simulink model "Appl_DrMotorAdjust_CtrlModel"  (R2018b)
settings: configuration reference "CodeConfig_10_ms" (kept outside this file)
undefined symbols (not defined in the file): CAL_HightMotorRunInterval_100ms, CAL_MotorDiffToStart_100ms, CAL_MotorStopTime_50ms, D_Relay_DownBackFault, D_Relay_UpFrontFault, D_ToleranceDistance, enSeatMoveCmd, FALSE, TRUE
libraries: DareLib x88, simulink x2
(part 1 of 3)
settings Model: Creator=Administrator  LastModifiedBy=Administrator
settings ConfigSetRef: SourceLocation=Base Workspace

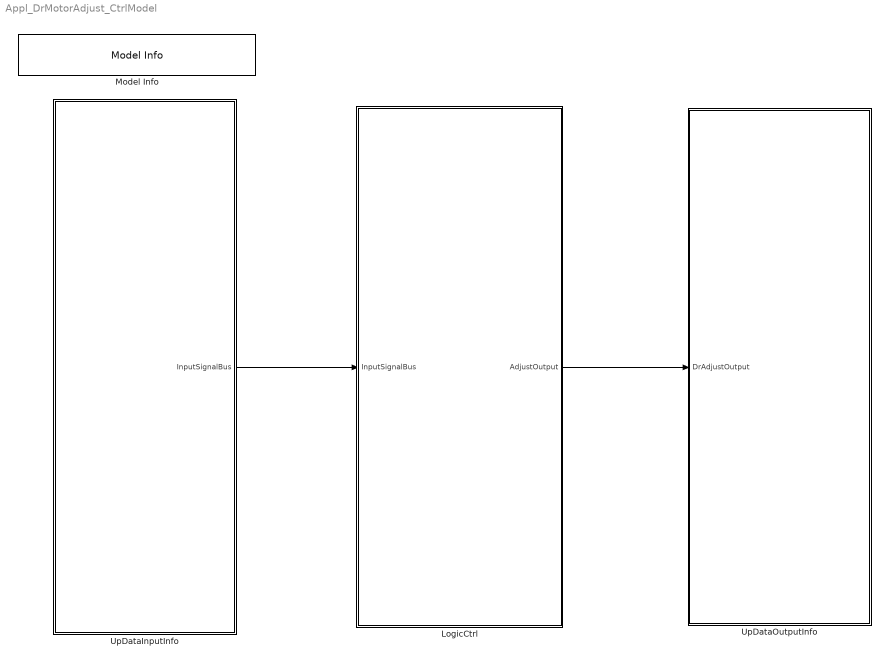
== system Appl_DrMotorAdjust_CtrlModel ==
  LogicCtrl : Subsystem  Priority=2  TreatAsAtomicUnit=on
      settings: RTWSystemCode=Nonreusable function  RTWFcnNameOpts=Use subsystem name
  Model Info : simulink/Model-Wide Utilities/Model Info  Frame=on  DisplayStringWithTags=Version：%<ModelVersion>  HorizontalTextAlignment=Center  LeftAlignmentValue=0.5
  UpDataInputInfo : Subsystem  Priority=1  TreatAsAtomicUnit=on
      settings: RTWSystemCode=Nonreusable function  RTWFcnNameOpts=Use subsystem name
  UpDataOutputInfo : Subsystem  Priority=3  TreatAsAtomicUnit=on
      settings: RTWSystemCode=Nonreusable function  RTWFcnNameOpts=Use subsystem name
  wires:
  UpDataInputInfo/1(InputSignalBus) -> LogicCtrl/1(InputSignalBus)
  LogicCtrl/1(AdjustOutput) -> UpDataOutputInfo/1(DrAdjustOutput)

== system Appl_DrMotorAdjust_CtrlModel/LogicCtrl ==
  InputSignalBus : Inport
  LocalAdjustCtrl : Subsystem  Description=调节逻辑处理
      settings: AttributesFormatString=%<Description>
  AdjustOutput : Outport
  wires:
  InputSignalBus/1 -> LocalAdjustCtrl/1(RteInputBus)  "RteInputBus"
  LocalAdjustCtrl/1(LocalAdjustCtrlOut) -> AdjustOutput/1

== system Appl_DrMotorAdjust_CtrlModel/UpDataInputInfo ==
  InputSignalProcess : Subsystem  Description=数据处理
      settings: AttributesFormatString=%<Description>  RTWSystemCode=Nonreusable function  RTWFcnNameOpts=Use subsystem name
  RTE : Subsystem  Description=接口自动生成  TreatAsAtomicUnit=on
      settings: AttributesFormatString=%<Description>  RTWSystemCode=Nonreusable function  RTWFcnNameOpts=Use subsystem name
  InputSignalBus : Outport
  wires:
  RTE/1(RTE_Signal) -> InputSignalProcess/1(Rte_SignalBus)
  InputSignalProcess/1(InputSignalBus) -> InputSignalBus/1

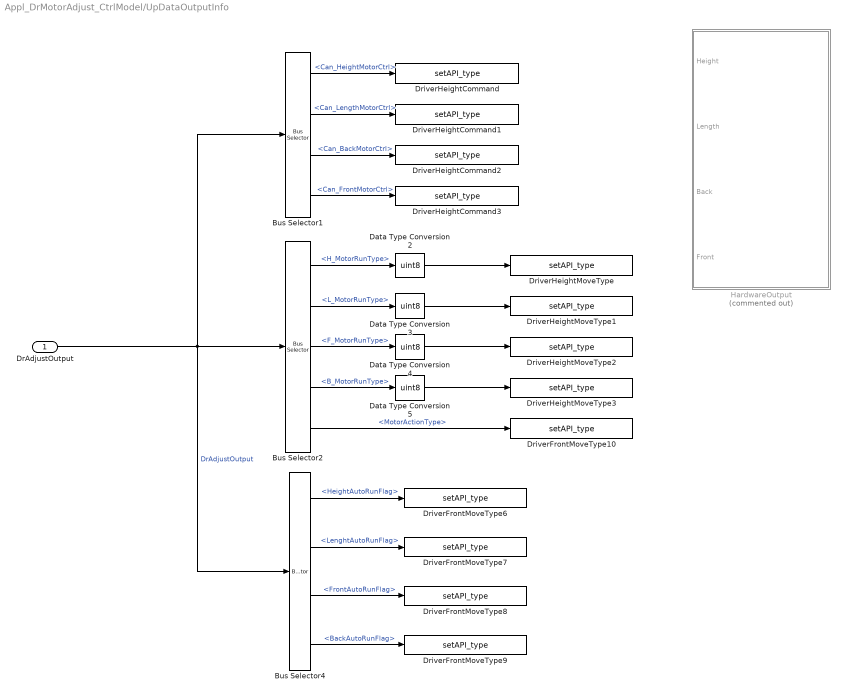
== system Appl_DrMotorAdjust_CtrlModel/UpDataOutputInfo ==
  DrAdjustOutput : Inport
  Bus Selector1 : BusSelector  OutputSignals=MotorCtrl.Can_HeightMotorCtrl,MotorCtrl.Can_LengthMotorCtrl,MotorCtrl.Can_BackMotorCtrl,MotorCtrl.Can_FrontMotorCtrl
  Bus Selector2 : BusSelector  OutputSignals=MotorRunType.H_MotorRunType,MotorRunType.L_MotorRunType,MotorRunType.F_MotorRunType,MotorRunType.B_MotorRunType,MotorReq.MotorActionType
  Bus Selector4 : BusSelector  OutputSignals=AutoRunFlag.HeightAutoRunFlag,AutoRunFlag.LenghtAutoRunFlag,AutoRunFlag.FrontAutoRunFlag,AutoRunFlag.BackAutoRunFlag
  Data Type Conversion{2..5} (4 alike) : DataTypeConversion  OutDataTypeStr=uint8
  DriverFrontMoveType10 : DareLib/Dare/setAPI_type  g_funcname=Rte_SetVfb_DrMoveType  g_param=""  g_type=uint8  g_enum=enSeatMotorRunTye  g_size=-1
      settings: AttributesFormatString=%<g_funcname>  SourceProductName=Dare Library
  DriverFrontMoveType6 : DareLib/Dare/setAPI_type  g_funcname=Rte_SetVfb_DrHeightAutoRunFlag  g_param=""  g_type=uint8  g_enum=enSeatAutoRunSts  g_size=-1
      settings: AttributesFormatString=%<g_funcname>  SourceProductName=Dare Library
  DriverFrontMoveType7 : DareLib/Dare/setAPI_type  g_funcname=Rte_SetVfb_DrLengthAutoRunFlag  g_param=""  g_type=uint8  g_enum=enSeatAutoRunSts  g_size=-1
      settings: AttributesFormatString=%<g_funcname>  SourceProductName=Dare Library
  DriverFrontMoveType8 : DareLib/Dare/setAPI_type  g_funcname=Rte_SetVfb_DrBackAutoRunFlag  g_param=""  g_type=uint8  g_enum=enSeatAutoRunSts  g_size=-1
      settings: AttributesFormatString=%<g_funcname>  SourceProductName=Dare Library
  DriverFrontMoveType9 : DareLib/Dare/setAPI_type  g_funcname=Rte_SetVfb_DrFrontAutoRunFlag  g_param=""  g_type=uint8  g_enum=enSeatAutoRunSts  g_size=-1
      settings: AttributesFormatString=%<g_funcname>  SourceProductName=Dare Library
  DriverHeightCommand : DareLib/Dare/setAPI_type  g_funcname=Rte_SetVfb_DrHeightMotorCmd  g_param=""  g_type=uint8  g_size=-1
      settings: AttributesFormatString=%<g_funcname>  SourceProductName=Dare Library
  DriverHeightCommand1 : DareLib/Dare/setAPI_type  g_funcname=Rte_SetVfb_DrLengthMotorCmd  g_param=""  g_type=uint8  g_size=-1
      settings: AttributesFormatString=%<g_funcname>  SourceProductName=Dare Library
  DriverHeightCommand2 : DareLib/Dare/setAPI_type  g_funcname=Rte_SetVfb_DrBackMotorCmd  g_param=""  g_type=uint8  g_size=-1
      settings: AttributesFormatString=%<g_funcname>  SourceProductName=Dare Library
  DriverHeightCommand3 : DareLib/Dare/setAPI_type  g_funcname=Rte_SetVfb_DrFrontMotorCmd  g_param=""  g_type=uint8  g_size=-1
      settings: AttributesFormatString=%<g_funcname>  SourceProductName=Dare Library
  DriverHeightMoveType : DareLib/Dare/setAPI_type  g_funcname=Rte_SetVfb_DrHeightMotorReason  g_param=""  g_type=uint8  g_size=-1
      settings: AttributesFormatString=%<g_funcname>  SourceProductName=Dare Library
  DriverHeightMoveType1 : DareLib/Dare/setAPI_type  g_funcname=Rte_SetVfb_DrLengthMotorReason  g_param=""  g_type=uint8  g_size=-1
      settings: AttributesFormatString=%<g_funcname>  SourceProductName=Dare Library
  DriverHeightMoveType2 : DareLib/Dare/setAPI_type  g_funcname=Rte_SetVfb_DrBackMotorReason  g_param=""  g_type=uint8  g_size=-1
      settings: AttributesFormatString=%<g_funcname>  SourceProductName=Dare Library
  DriverHeightMoveType3 : DareLib/Dare/setAPI_type  g_funcname=Rte_SetVfb_DrFrontMotorReason  g_param=""  g_type=uint8  g_size=-1
      settings: AttributesFormatString=%<g_funcname>  SourceProductName=Dare Library
  HardwareOutput : Subsystem  Commented=on
  wires:
  DrAdjustOutput/1 -> Bus Selector4/1, Bus Selector1/1, Bus Selector2/1  "DrAdjustOutput"
  Data Type Conversion2/1 -> DriverHeightMoveType/1
  Data Type Conversion3/1 -> DriverHeightMoveType1/1
  Data Type Conversion4/1 -> DriverHeightMoveType2/1
  Data Type Conversion5/1 -> DriverHeightMoveType3/1
  Bus Selector1/1 -> DriverHeightCommand/1  "<Can_HeightMotorCtrl>"
  Bus Selector1/2 -> DriverHeightCommand1/1  "<Can_LengthMotorCtrl>"
  Bus Selector1/3 -> DriverHeightCommand2/1  "<Can_BackMotorCtrl>"
  Bus Selector1/4 -> DriverHeightCommand3/1  "<Can_FrontMotorCtrl>"
  Bus Selector2/1 -> Data Type Conversion2/1  "<H_MotorRunType>"
  Bus Selector2/2 -> Data Type Conversion3/1  "<L_MotorRunType>"
  Bus Selector2/3 -> Data Type Conversion4/1  "<F_MotorRunType>"
  Bus Selector2/4 -> Data Type Conversion5/1  "<B_MotorRunType>"
  Bus Selector2/5 -> DriverFrontMoveType10/1  "<MotorActionType>"
  Bus Selector4/4 -> DriverFrontMoveType9/1  "<BackAutoRunFlag>"
  Bus Selector4/3 -> DriverFrontMoveType8/1  "<FrontAutoRunFlag>"
  Bus Selector4/2 -> DriverFrontMoveType7/1  "<LenghtAutoRunFlag>"
  Bus Selector4/1 -> DriverFrontMoveType6/1  "<HeightAutoRunFlag>"

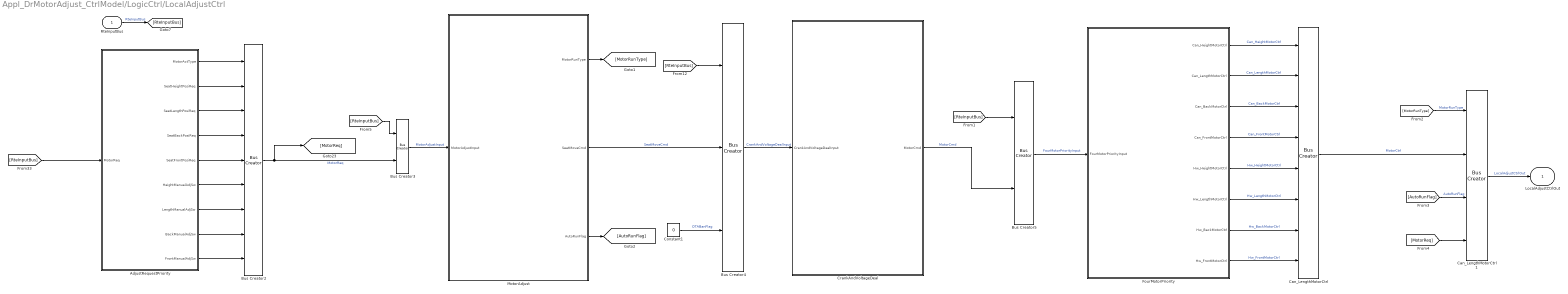
== system Appl_DrMotorAdjust_CtrlModel/LogicCtrl/LocalAdjustCtrl ==
  RteInputBus : Inport
  AdjustRequestPriority : Subsystem  Description=电机运动请求优先级处理
      settings: AttributesFormatString=%<Description>
      mask Display: image('优先级.png');
  Bus Creator2 : BusCreator  Inputs=9
  Bus Creator3 : BusCreator  Inputs=2
  Bus Creator4 : BusCreator  Inputs=3
  Bus Creator5 : BusCreator  Inputs=2
  Can_LengthMotorCtrl : BusCreator  Inputs=8
  Can_LengthMotorCtrl1 : BusCreator  Inputs=4
  Constant1 : Constant  Value=0
  CrankAndVoltageDeal : Subsystem  Description=CRANK卸荷和电压限制处理
      settings: AttributesFormatString=%<Description>
      mask Display: image('卸荷.png');
  FourMotorPriority : Subsystem  Description=四向调节电机运动优先级
      settings: AttributesFormatString=%<Description>
      mask Display: image('电机优先级.png');
  MotorAdjust : Subsystem  Description=四向电机调节
      settings: AttributesFormatString=%<Description>
      mask Display: image('电机调节.png');
  LocalAdjustCtrlOut : Outport
  wires:
  MotorAdjust/3(AutoRunFlag) -> [AutoRunFlag]
  [RteInputBus] -> Bus Creator4/1
  RteInputBus/1 -> [RteInputBus]  "RteInputBus"
  [RteInputBus] -> AdjustRequestPriority/1(MotorReq)
  Bus Creator2/1 -> [MotorReq], Bus Creator3/2  "MotorReq"
  [RteInputBus] -> Bus Creator3/1
  Bus Creator3/1 -> MotorAdjust/1(MotorAdjustInput)  "MotorAdjustInput"
  Constant1/1 -> Bus Creator4/3  "OTABanFlag"
  MotorAdjust/2(SeatMoveCmd) -> Bus Creator4/2  "SeatMoveCmd"
  Bus Creator4/1 -> CrankAndVoltageDeal/1(CrankAndVoltageDealInput)  "CrankAndVoltageDealInput"
  CrankAndVoltageDeal/1(MotorCmd) -> Bus Creator5/2  "MotorCmd"
  [RteInputBus] -> Bus Creator5/1
  Bus Creator5/1 -> FourMotorPriority/1(FourMotorPriorityInput)  "FourMotorPriorityInput"
  MotorAdjust/1(MotorRunType) -> [MotorRunType]
  [MotorRunType] -> Can_LengthMotorCtrl1/1  "MotorRunType"
  [AutoRunFlag] -> Can_LengthMotorCtrl1/3  "AutoRunFlag"
  Can_LengthMotorCtrl/1 -> Can_LengthMotorCtrl1/2  "MotorCtrl"
  Can_LengthMotorCtrl1/1 -> LocalAdjustCtrlOut/1  "LocalAdjustCtrlOut"
  [MotorReq] -> Can_LengthMotorCtrl1/4
  AdjustRequestPriority/1(MotorActType) -> Bus Creator2/1
  AdjustRequestPriority/2(SeatHeightPosiReq) -> Bus Creator2/2
  AdjustRequestPriority/3(SeatLengthPosiReq) -> Bus Creator2/3
  AdjustRequestPriority/4(SeatBackPosiReq) -> Bus Creator2/4
  AdjustRequestPriority/5(SeatFrontPosiReq) -> Bus Creator2/5
  AdjustRequestPriority/6(HeightManualAdjSw) -> Bus Creator2/6
  AdjustRequestPriority/7(LengthManualAdjSw) -> Bus Creator2/7
  AdjustRequestPriority/8(BackManualAdjSw) -> Bus Creator2/8
  AdjustRequestPriority/9(FrontManualAdjSw) -> Bus Creator2/9
  FourMotorPriority/1(Can_HeightMotorCtrl) -> Can_LengthMotorCtrl/1  "Can_HeightMotorCtrl"
  FourMotorPriority/2(Can_LengthMotorCtrl) -> Can_LengthMotorCtrl/2  "Can_LengthMotorCtrl"
  FourMotorPriority/3(Can_BackMotorCtrl) -> Can_LengthMotorCtrl/3  "Can_BackMotorCtrl"
  FourMotorPriority/4(Can_FrontMotorCtrl) -> Can_LengthMotorCtrl/4  "Can_FrontMotorCtrl"
  FourMotorPriority/5(Hw_HeightMotorCtrl) -> Can_LengthMotorCtrl/5  "Hw_HeightMotorCtrl"
  FourMotorPriority/6(Hw_LengthMotorCtrl) -> Can_LengthMotorCtrl/6  "Hw_LengthMotorCtrl"
  FourMotorPriority/7(Hw_BackMotorCtrl) -> Can_LengthMotorCtrl/7  "Hw_BackMotorCtrl"
  FourMotorPriority/8(Hw_FrontMotorCtrl) -> Can_LengthMotorCtrl/8  "Hw_FrontMotorCtrl"

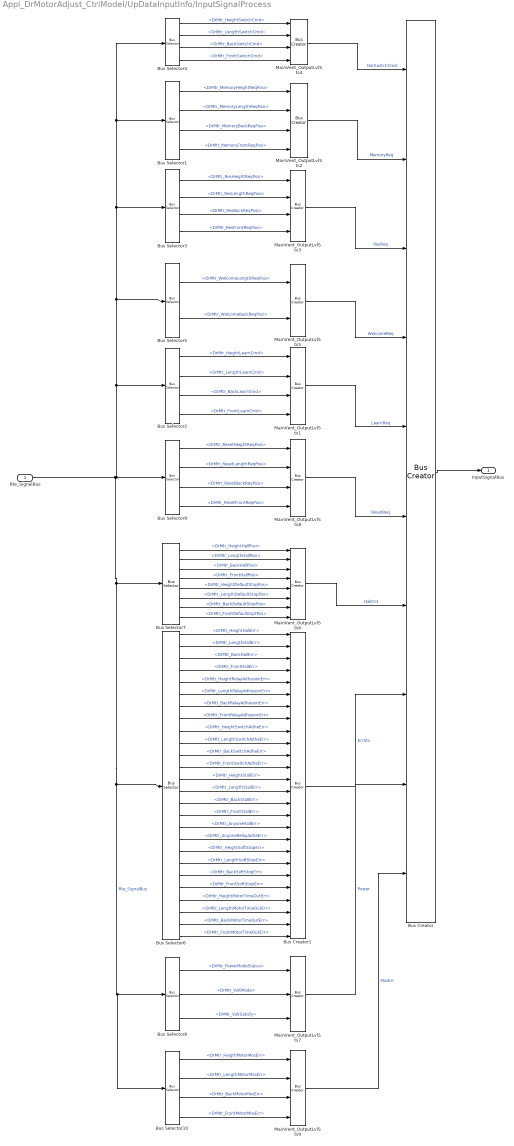
== system Appl_DrMotorAdjust_CtrlModel/UpDataInputInfo/InputSignalProcess ==
  Rte_SignalBus : Inport
  Bus Creator : BusCreator  Inputs=10
  Bus Creator1 : BusCreator  Inputs=26
  Bus Selector1 : BusSelector  OutputSignals=DrMtr_MemoryHeightReqPosi,DrMtr_MemoryLengthReqPosi,DrMtr_MemoryBackReqPosi,DrMtr_MemoryFrontReqPosi
  Bus Selector10 : BusSelector  OutputSignals=DrMtr_HeigthMotorMosErr,DrMtr_LengthMotorMosErr,DrMtr_BackMotorMosErr,DrMtr_FrontMotorMosErr
  Bus Selector2 : BusSelector  OutputSignals=DrMtr_HeightLearnCmd,DrMtr_LengthLearnCmd,DrMtr_BackLearnCmd,DrMtr_FrontLearnCmd
  Bus Selector3 : BusSelector  OutputSignals=DrMtr_ResHeightReqPosi,DrMtr_ResLengthReqPosi,DrMtr_ResBackReqPosi,DrMtr_ResFrontReqPosi
  Bus Selector4 : BusSelector  OutputSignals=DrMtr_HeightSwitchCmd,DrMtr_LengthSwitchCmd,DrMtr_BackSwitchCmd,DrMtr_FrontSwitchCmd
  Bus Selector5 : BusSelector  OutputSignals=DrMtr_WelcomeLengthReqPosi,DrMtr_WelcomeBackReqPosi
  Bus Selector6 : BusSelector  OutputSignals=DrMtr_HeightHallErr,DrMtr_LengthHallErr,DrMtr_BackHallErr,DrMtr_FrontHallErr,DrMtr_HeightRelayAdhesionErr,DrMtr_LengthRelayAdhesionErr,DrMtr_BackRelayAdhesionErr,DrMtr_FrontRelayAdhesionErr,DrMtr_HeightSwitchAdheErr,DrMtr_LengthSwitchAdheErr,DrMtr_BackSwitchAdheErr,DrMtr_FrontSwitchAdheErr,DrMtr_HeightStallErr,DrMtr_LengthStallErr,DrMtr_BackStallErr,DrMtr_FrontStallErr,DrMtr_AnyoneHallErr,DrMtr_AnyoneRelayAdheErr,DrMtr_HeightSoftStopErr,DrMtr_LengthSoftStopErr,DrMtr_BackSoftStopErr,DrMtr_FrontSoftStopErr,DrMtr_HeightMotorTimeOutErr,DrMtr_LengthMotorTimeOutErr,DrMtr_BackMotorTimeOutErr,DrMtr_FrontMotorTimeOutErr
  Bus Selector7 : BusSelector  OutputSignals=DrMtr_HeightHallPosi,DrMtr_LengthHallPosi,DrMtr_BackHallPosi,DrMtr_FrontHallPosi,DrMtr_HeightDefaultStopPos,DrMtr_LengthDefaultStopPos,DrMtr_BackDefaultStopPos,DrMtr_FrontDefaulStoptPos
  Bus Selector8 : BusSelector  OutputSignals=DrMtr_PowerModeStatus,DrMtr_VoltMode,DrMtr_VoltSatisfy
  Bus Selector9 : BusSelector  OutputSignals=DrMtr_ResetHeightReqPosi,DrMtr_ResetLengthReqPosi,DrMtr_ResetBackReqPosi,DrMtr_ResetFrontReqPosi
  MainVent_OutputLvlSts{1..4,8..9} (6 alike) : BusCreator  Inputs=4
  MainVent_OutputLvlSts5 : BusCreator  Inputs=2
  MainVent_OutputLvlSts6 : BusCreator  Inputs=8
  MainVent_OutputLvlSts7 : BusCreator  Inputs=3
  InputSignalBus : Outport
  wires:
  Bus Selector4/1 -> MainVent_OutputLvlSts4/1  "<DrMtr_HeightSwitchCmd>"
  Bus Selector4/2 -> MainVent_OutputLvlSts4/2  "<DrMtr_LengthSwitchCmd>"
  Bus Selector4/3 -> MainVent_OutputLvlSts4/3  "<DrMtr_BackSwitchCmd>"
  Bus Selector4/4 -> MainVent_OutputLvlSts4/4  "<DrMtr_FrontSwitchCmd>"
  Bus Selector1/1 -> MainVent_OutputLvlSts2/1  "<DrMtr_MemoryHeightReqPosi>"
  Bus Selector1/2 -> MainVent_OutputLvlSts2/2  "<DrMtr_MemoryLengthReqPosi>"
  Bus Selector1/3 -> MainVent_OutputLvlSts2/3  "<DrMtr_MemoryBackReqPosi>"
  Bus Selector1/4 -> MainVent_OutputLvlSts2/4  "<DrMtr_MemoryFrontReqPosi>"
  Bus Selector3/3 -> MainVent_OutputLvlSts3/3  "<DrMtr_ResBackReqPosi>"
  Bus Selector3/2 -> MainVent_OutputLvlSts3/2  "<DrMtr_ResLengthReqPosi>"
  Bus Selector3/4 -> MainVent_OutputLvlSts3/4  "<DrMtr_ResFrontReqPosi>"
  Bus Selector3/1 -> MainVent_OutputLvlSts3/1  "<DrMtr_ResHeightReqPosi>"
  Bus Selector7/1 -> MainVent_OutputLvlSts6/1  "<DrMtr_HeightHallPosi>"
  Bus Selector7/2 -> MainVent_OutputLvlSts6/2  "<DrMtr_LengthHallPosi>"
  Bus Selector7/3 -> MainVent_OutputLvlSts6/3  "<DrMtr_BackHallPosi>"
  Bus Selector7/4 -> MainVent_OutputLvlSts6/4  "<DrMtr_FrontHallPosi>"
  Bus Selector7/5 -> MainVent_OutputLvlSts6/5  "<DrMtr_HeightDefaultStopPos>"
  Bus Selector7/6 -> MainVent_OutputLvlSts6/6  "<DrMtr_LengthDefaultStopPos>"
  Bus Selector7/7 -> MainVent_OutputLvlSts6/7  "<DrMtr_BackDefaultStopPos>"
  Bus Selector2/1 -> MainVent_OutputLvlSts1/1  "<DrMtr_HeightLearnCmd>"
  Bus Selector2/2 -> MainVent_OutputLvlSts1/2  "<DrMtr_LengthLearnCmd>"
  Bus Selector8/2 -> MainVent_OutputLvlSts7/2  "<DrMtr_VoltMode>"
  Bus Selector8/1 -> MainVent_OutputLvlSts7/1  "<DrMtr_PowerModeStatus>"
  Bus Selector8/3 -> MainVent_OutputLvlSts7/3  "<DrMtr_VoltSatisfy>"
  MainVent_OutputLvlSts7/1 -> Bus Creator/9  "Power"
  MainVent_OutputLvlSts4/1 -> Bus Creator/1  "HarSwitchCmd"
  MainVent_OutputLvlSts2/1 -> Bus Creator/2  "MemoryReq"
  Bus Creator1/1 -> Bus Creator/8  "ErrSts"
  MainVent_OutputLvlSts3/1 -> Bus Creator/3  "ResReq"
  MainVent_OutputLvlSts5/1 -> Bus Creator/4  "WelcomeReq"
  MainVent_OutputLvlSts1/1 -> Bus Creator/5  "LearnReq"
  MainVent_OutputLvlSts6/1 -> Bus Creator/7  "HallCnt"
  Bus Selector6/1 -> Bus Creator1/1  "<DrMtr_HeightHallErr>"
  Bus Selector6/2 -> Bus Creator1/2  "<DrMtr_LengthHallErr>"
  Bus Selector6/3 -> Bus Creator1/3  "<DrMtr_BackHallErr>"
  Bus Selector6/4 -> Bus Creator1/4  "<DrMtr_FrontHallErr>"
  Bus Selector6/5 -> Bus Creator1/5  "<DrMtr_HeightRelayAdhesionErr>"
  Bus Selector6/6 -> Bus Creator1/6  "<DrMtr_LengthRelayAdhesionErr>"
  Bus Selector6/7 -> Bus Creator1/7  "<DrMtr_BackRelayAdhesionErr>"
  Bus Selector6/8 -> Bus Creator1/8  "<DrMtr_FrontRelayAdhesionErr>"
  Bus Selector6/9 -> Bus Creator1/9  "<DrMtr_HeightSwitchAdheErr>"
  Bus Selector6/10 -> Bus Creator1/10  "<DrMtr_LengthSwitchAdheErr>"
  Bus Selector6/11 -> Bus Creator1/11  "<DrMtr_BackSwitchAdheErr>"
  Bus Selector6/12 -> Bus Creator1/12  "<DrMtr_FrontSwitchAdheErr>"
  Bus Selector6/13 -> Bus Creator1/13  "<DrMtr_HeightStallErr>"
  Bus Selector6/14 -> Bus Creator1/14  "<DrMtr_LengthStallErr>"
  Bus Selector6/15 -> Bus Creator1/15  "<DrMtr_BackStallErr>"
  Bus Selector6/16 -> Bus Creator1/16  "<DrMtr_FrontStallErr>"
  Bus Selector6/17 -> Bus Creator1/17  "<DrMtr_AnyoneHallErr>"
  Bus Selector6/18 -> Bus Creator1/18  "<DrMtr_AnyoneRelayAdheErr>"
  Bus Selector6/19 -> Bus Creator1/19  "<DrMtr_HeightSoftStopErr>"
  Bus Selector6/20 -> Bus Creator1/20  "<DrMtr_LengthSoftStopErr>"
  Bus Selector6/21 -> Bus Creator1/21  "<DrMtr_BackSoftStopErr>"
  Bus Selector6/22 -> Bus Creator1/22  "<DrMtr_FrontSoftStopErr>"
  Bus Selector6/23 -> Bus Creator1/23  "<DrMtr_HeightMotorTimeOutErr>"
  Bus Selector6/24 -> Bus Creator1/24  "<DrMtr_LengthMotorTimeOutErr>"
  Bus Selector6/25 -> Bus Creator1/25  "<DrMtr_BackMotorTimeOutErr>"
  Bus Selector6/26 -> Bus Creator1/26  "<DrMtr_FrontMotorTimeOutErr>"
  Bus Selector5/1 -> MainVent_OutputLvlSts5/1  "<DrMtr_WelcomeLengthReqPosi>"
  Bus Selector5/2 -> MainVent_OutputLvlSts5/2  "<DrMtr_WelcomeBackReqPosi>"
  Bus Selector2/3 -> MainVent_OutputLvlSts1/3  "<DrMtr_BackLearnCmd>"
  Bus Selector2/4 -> MainVent_OutputLvlSts1/4  "<DrMtr_FrontLearnCmd>"
  Bus Selector9/4 -> MainVent_OutputLvlSts8/4  "<DrMtr_ResetFrontReqPosi>"
  Bus Selector9/3 -> MainVent_OutputLvlSts8/3  "<DrMtr_ResetBackReqPosi>"
  MainVent_OutputLvlSts8/1 -> Bus Creator/6  "ResetReq"
  Bus Selector9/2 -> MainVent_OutputLvlSts8/2  "<DrMtr_ResetLengthReqPosi>"
  Rte_SignalBus/1 -> Bus Selector9/1, Bus Selector3/1, Bus Selector4/1, Bus Selector1/1, Bus Selector5/1, Bus Selector2/1, Bus Selector7/1, Bus Selector10/1, Bus Selector8/1, Bus Selector6/1  "Rte_SignalBus"
  Bus Selector9/1 -> MainVent_OutputLvlSts8/1  "<DrMtr_ResetHeightReqPosi>"
  Bus Selector7/8 -> MainVent_OutputLvlSts6/8  "<DrMtr_FrontDefaulStoptPos>"
  Bus Creator/1 -> InputSignalBus/1
  Bus Selector10/3 -> MainVent_OutputLvlSts9/3  "<DrMtr_BackMotorMosErr>"
  Bus Selector10/1 -> MainVent_OutputLvlSts9/1  "<DrMtr_HeigthMotorMosErr>"
  Bus Selector10/2 -> MainVent_OutputLvlSts9/2  "<DrMtr_LengthMotorMosErr>"
  Bus Selector10/4 -> MainVent_OutputLvlSts9/4  "<DrMtr_FrontMotorMosErr>"
  MainVent_OutputLvlSts9/1 -> Bus Creator/10  "MosErr"

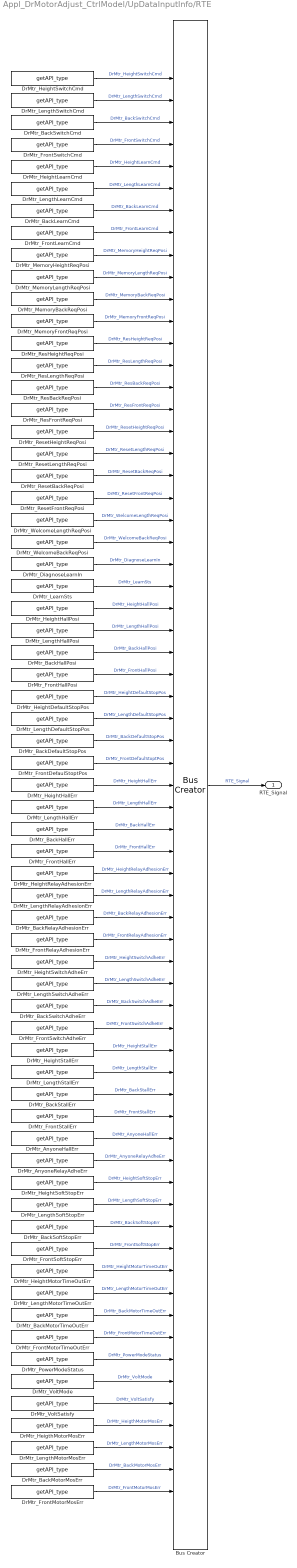
== system Appl_DrMotorAdjust_CtrlModel/UpDataInputInfo/RTE ==
  Bus Creator : BusCreator  Inputs=65
  DrMtr_AnyoneHallErr : DareLib/Dare/getAPI_type  g_funcname=Rte_GetVfb_DrAnyoneHallErr  g_param=""  g_type=uint8  g_size=-1
      settings: AttributesFormatString=%<g_funcname>  SourceProductName=Dare Library
  DrMtr_AnyoneRelayAdheErr : DareLib/Dare/getAPI_type  g_funcname=Rte_GetVfb_DrAnyoneRelayAdheErr  g_param=""  g_type=uint8  g_size=-1
      settings: AttributesFormatString=%<g_funcname>  SourceProductName=Dare Library
  DrMtr_BackDefaultStopPos : DareLib/Dare/getAPI_type  g_funcname=Cdd_GetMotorHardStop  g_param=EN_DriverBack  g_type=uint16  g_size=-1
      settings: AttributesFormatString=%<g_funcname>  SourceProductName=Dare Library
  DrMtr_BackHallErr : DareLib/Dare/getAPI_type  g_funcname=Rte_GetVfb_DrBackHallErr  g_param=""  g_type=uint8  g_size=-1
      settings: AttributesFormatString=%<g_funcname>  SourceProductName=Dare Library
  DrMtr_BackHallPosi : DareLib/Dare/getAPI_type  g_funcname=Cdd_GetCurrentHallCnt  g_param=EN_DriverBack  g_type=uint16  g_size=-1
      settings: AttributesFormatString=%<g_funcname>  SourceProductName=Dare Library
  DrMtr_BackLearnCmd : DareLib/Dare/getAPI_type  g_funcname=Rte_GetVfb_DrBackLearnCmd  g_param=""  g_type=uint8  g_size=-1
      settings: AttributesFormatString=%<g_funcname>  SourceProductName=Dare Library
  DrMtr_BackMotorMosErr : DareLib/Dare/getAPI_type  g_funcname=Srvl_Tle9210x_GetMotorErr  g_param=EN_SEAT_DRV_BACK  g_type=uint8  g_enum=enMosErrSts  g_size=-1
      settings: AttributesFormatString=%<g_funcname>  SourceProductName=Dare Library
  DrMtr_BackMotorTimeOutErr : DareLib/Dare/getAPI_type  g_funcname=Rte_GetVfb_DrBackMotorTimeOutErr  g_param=""  g_type=uint8  g_size=-1
      settings: AttributesFormatString=%<g_funcname>  SourceProductName=Dare Library
  DrMtr_BackRelayAdhesionErr : DareLib/Dare/getAPI_type  g_funcname=Rte_GetVfb_DrBackRelayAdheErr  g_param=""  g_type=uint8  g_size=-1
      settings: AttributesFormatString=%<g_funcname>  SourceProductName=Dare Library
  DrMtr_BackSoftStopErr : DareLib/Dare/getAPI_type  g_funcname=Rte_GetVfb_DrBackSoftStopErr  g_param=""  g_type=uint8  g_size=-1
      settings: AttributesFormatString=%<g_funcname>  SourceProductName=Dare Library
  DrMtr_BackStallErr : DareLib/Dare/getAPI_type  g_funcname=Rte_GetVfb_DrBackStallErr  g_param=""  g_type=uint8  g_size=-1
      settings: AttributesFormatString=%<g_funcname>  SourceProductName=Dare Library
  DrMtr_BackSwitchAdheErr : DareLib/Dare/getAPI_type  g_funcname=Rte_GetVfb_DrBackSwitchAdheErr  g_param=""  g_type=uint8  g_size=-1
      settings: AttributesFormatString=%<g_funcname>  SourceProductName=Dare Library
  DrMtr_BackSwitchCmd : DareLib/Dare/getAPI_type  g_funcname=Rte_GetVfb_DrBackSwitchCmd  g_param=""  g_type=uint8  g_size=-1
      settings: AttributesFormatString=%<g_funcname>  SourceProductName=Dare Library
  DrMtr_DiagnoseLearnIn : DareLib/Dare/getAPI_type  g_funcname=Rte_GetVfb_DrLearnEnable  g_param=""  g_type=uint8  g_size=-1
      settings: AttributesFormatString=%<g_funcname>  SourceProductName=Dare Library
  DrMtr_FrontDefaulStoptPos : DareLib/Dare/getAPI_type  g_funcname=Cdd_GetMotorHardStop  g_param=EN_DriverFront  g_type=uint16  g_size=-1
      settings: AttributesFormatString=%<g_funcname>  SourceProductName=Dare Library
  DrMtr_FrontHallErr : DareLib/Dare/getAPI_type  g_funcname=Rte_GetVfb_DrFrontHallErr  g_param=""  g_type=uint8  g_size=-1
      settings: AttributesFormatString=%<g_funcname>  SourceProductName=Dare Library
  DrMtr_FrontHallPosi : DareLib/Dare/getAPI_type  g_funcname=Cdd_GetCurrentHallCnt  g_param=EN_DriverFront  g_type=uint16  g_size=-1
      settings: AttributesFormatString=%<g_funcname>  SourceProductName=Dare Library
  DrMtr_FrontLearnCmd : DareLib/Dare/getAPI_type  g_funcname=Rte_GetVfb_DrFrontLearnCmd  g_param=""  g_type=uint8  g_size=-1
      settings: AttributesFormatString=%<g_funcname>  SourceProductName=Dare Library
  DrMtr_FrontMotorMosErr : DareLib/Dare/getAPI_type  g_funcname=Srvl_Tle9210x_GetMotorErr  g_param=EN_SEAT_DRV_FRONT  g_type=uint8  g_enum=enMosErrSts  g_size=-1
      settings: AttributesFormatString=%<g_funcname>  SourceProductName=Dare Library
  DrMtr_FrontMotorTimeOutErr : DareLib/Dare/getAPI_type  g_funcname=Rte_GetVfb_DrFrontMotorTimeOutErr  g_param=""  g_type=uint8  g_size=-1
      settings: AttributesFormatString=%<g_funcname>  SourceProductName=Dare Library
  DrMtr_FrontRelayAdhesionErr : DareLib/Dare/getAPI_type  g_funcname=Rte_GetVfb_DrFrontRelayAdheErr  g_param=""  g_type=uint8  g_size=-1
      settings: AttributesFormatString=%<g_funcname>  SourceProductName=Dare Library
  DrMtr_FrontSoftStopErr : DareLib/Dare/getAPI_type  g_funcname=Rte_GetVfb_DrFrontSoftStopErr  g_param=""  g_type=uint8  g_size=-1
      settings: AttributesFormatString=%<g_funcname>  SourceProductName=Dare Library
  DrMtr_FrontStallErr : DareLib/Dare/getAPI_type  g_funcname=Rte_GetVfb_DrFrontStallErr  g_param=""  g_type=uint8  g_size=-1
      settings: AttributesFormatString=%<g_funcname>  SourceProductName=Dare Library
  DrMtr_FrontSwitchAdheErr : DareLib/Dare/getAPI_type  g_funcname=Rte_GetVfb_DrFrontSwitchAdheErr  g_param=""  g_type=uint8  g_size=-1
      settings: AttributesFormatString=%<g_funcname>  SourceProductName=Dare Library
  DrMtr_FrontSwitchCmd : DareLib/Dare/getAPI_type  g_funcname=Rte_GetVfb_DrFrontSwitchCmd  g_param=""  g_type=uint8  g_size=-1
      settings: AttributesFormatString=%<g_funcname>  SourceProductName=Dare Library
  DrMtr_HeightDefaultStopPos : DareLib/Dare/getAPI_type  g_funcname=Cdd_GetMotorHardStop  g_param=EN_DriverHeight  g_type=uint16  g_size=-1
      settings: AttributesFormatString=%<g_funcname>  SourceProductName=Dare Library
  DrMtr_HeightHallErr : DareLib/Dare/getAPI_type  g_funcname=Rte_GetVfb_DrHeightHallErr  g_param=""  g_type=uint8  g_size=-1
      settings: AttributesFormatString=%<g_funcname>  SourceProductName=Dare Library
  DrMtr_HeightHallPosi : DareLib/Dare/getAPI_type  g_funcname=Cdd_GetCurrentHallCnt  g_param=EN_DriverHeight  g_type=uint16  g_size=-1
      settings: AttributesFormatString=%<g_funcname>  SourceProductName=Dare Library
  DrMtr_HeightLearnCmd : DareLib/Dare/getAPI_type  g_funcname=Rte_GetVfb_DrHeightLearnCmd  g_param=""  g_type=uint8  g_size=-1
      settings: AttributesFormatString=%<g_funcname>  SourceProductName=Dare Library
  DrMtr_HeightMotorTimeOutErr : DareLib/Dare/getAPI_type  g_funcname=Rte_GetVfb_DrHeightMotorTimeOutErr  g_param=""  g_type=uint8  g_size=-1
      settings: AttributesFormatString=%<g_funcname>  SourceProductName=Dare Library
  DrMtr_HeightRelayAdhesionErr : DareLib/Dare/getAPI_type  g_funcname=Rte_GetVfb_DrHeightRelayAdheErr  g_param=""  g_type=uint8  g_size=-1
      settings: AttributesFormatString=%<g_funcname>  SourceProductName=Dare Library
  DrMtr_HeightSoftStopErr : DareLib/Dare/getAPI_type  g_funcname=Rte_GetVfb_DrLengthSoftStopErr  g_param=""  g_type=uint8  g_size=-1
      settings: AttributesFormatString=%<g_funcname>  SourceProductName=Dare Library
  DrMtr_HeightStallErr : DareLib/Dare/getAPI_type  g_funcname=Rte_GetVfb_DrHeightStallErr  g_param=""  g_type=uint8  g_size=-1
      settings: AttributesFormatString=%<g_funcname>  SourceProductName=Dare Library
  DrMtr_HeightSwitchAdheErr : DareLib/Dare/getAPI_type  g_funcname=Rte_GetVfb_DrHeightSwitchAdheErr  g_param=""  g_type=uint8  g_size=-1
      settings: AttributesFormatString=%<g_funcname>  SourceProductName=Dare Library
  DrMtr_HeightSwitchCmd : DareLib/Dare/getAPI_type  g_funcname=Rte_GetVfb_DrHeightSwitchCmd  g_param=""  g_type=uint8  g_size=-1
      settings: AttributesFormatString=%<g_funcname>  SourceProductName=Dare Library
  DrMtr_HeigthMotorMosErr : DareLib/Dare/getAPI_type  g_funcname=Srvl_Tle9210x_GetMotorErr  g_param=EN_SEAT_DRV_HEIGHT  g_type=uint8  g_enum=enMosErrSts  g_size=-1
      settings: AttributesFormatString=%<g_funcname>  SourceProductName=Dare Library
  DrMtr_LearnSts : DareLib/Dare/getAPI_type  g_funcname=Rte_GetVfb_DrLearnSts  g_param=""  g_type=uint8  g_size=-1
      settings: AttributesFormatString=%<g_funcname>  SourceProductName=Dare Library
  DrMtr_LengthDefaultStopPos : DareLib/Dare/getAPI_type  g_funcname=Cdd_GetMotorHardStop  g_param=EN_DriverLength  g_type=uint16  g_size=-1
      settings: AttributesFormatString=%<g_funcname>  SourceProductName=Dare Library
  DrMtr_LengthHallErr : DareLib/Dare/getAPI_type  g_funcname=Rte_GetVfb_DrLengthHallErr  g_param=""  g_type=uint8  g_size=-1
      settings: AttributesFormatString=%<g_funcname>  SourceProductName=Dare Library
  DrMtr_LengthHallPosi : DareLib/Dare/getAPI_type  g_funcname=Cdd_GetCurrentHallCnt  g_param=EN_DriverLength  g_type=uint16  g_size=-1
      settings: AttributesFormatString=%<g_funcname>  SourceProductName=Dare Library
  DrMtr_LengthLearnCmd : DareLib/Dare/getAPI_type  g_funcname=Rte_GetVfb_DrLengthLearnCmd  g_param=""  g_type=uint8  g_size=-1
      settings: AttributesFormatString=%<g_funcname>  SourceProductName=Dare Library
  DrMtr_LengthMotorMosErr : DareLib/Dare/getAPI_type  g_funcname=Srvl_Tle9210x_GetMotorErr  g_param=EN_SEAT_DRV_LENGTH  g_type=uint8  g_enum=enMosErrSts  g_size=-1
      settings: AttributesFormatString=%<g_funcname>  SourceProductName=Dare Library
  DrMtr_LengthMotorTimeOutErr : DareLib/Dare/getAPI_type  g_funcname=Rte_GetVfb_DrLengthMotorTimeOutErr  g_param=""  g_type=uint8  g_size=-1
      settings: AttributesFormatString=%<g_funcname>  SourceProductName=Dare Library
  DrMtr_LengthRelayAdhesionErr : DareLib/Dare/getAPI_type  g_funcname=Rte_GetVfb_DrLengthRelayAdheErr  g_param=""  g_type=uint8  g_size=-1
      settings: AttributesFormatString=%<g_funcname>  SourceProductName=Dare Library
  DrMtr_LengthSoftStopErr : DareLib/Dare/getAPI_type  g_funcname=Rte_GetVfb_DrHeightSoftStopErr  g_param=""  g_type=uint8  g_size=-1
      settings: AttributesFormatString=%<g_funcname>  SourceProductName=Dare Library
  DrMtr_LengthStallErr : DareLib/Dare/getAPI_type  g_funcname=Rte_GetVfb_DrLengthStallErr  g_param=""  g_type=uint8  g_size=-1
      settings: AttributesFormatString=%<g_funcname>  SourceProductName=Dare Library
  DrMtr_LengthSwitchAdheErr : DareLib/Dare/getAPI_type  g_funcname=Rte_GetVfb_DrLengthSwitchAdheErr  g_param=""  g_type=uint8  g_size=-1
      settings: AttributesFormatString=%<g_funcname>  SourceProductName=Dare Library
  DrMtr_LengthSwitchCmd : DareLib/Dare/getAPI_type  g_funcname=Rte_GetVfb_DrLengthSwitchCmd  g_param=""  g_type=uint8  g_size=-1
      settings: AttributesFormatString=%<g_funcname>  SourceProductName=Dare Library
  DrMtr_MemoryBackReqPosi : DareLib/Dare/getAPI_type  g_funcname=Rte_GetVfb_DrMemBackReqPosi  g_param=""  g_type=uint16  g_size=-1
      settings: AttributesFormatString=%<g_funcname>  SourceProductName=Dare Library
  DrMtr_MemoryFrontReqPosi : DareLib/Dare/getAPI_type  g_funcname=Rte_GetVfb_DrMemFrontReqPosi  g_param=""  g_type=uint16  g_size=-1
      settings: AttributesFormatString=%<g_funcname>  SourceProductName=Dare Library
  DrMtr_MemoryHeightReqPosi : DareLib/Dare/getAPI_type  g_funcname=Rte_GetVfb_DrMemHeightReqPosi  g_param=""  g_type=uint16  g_size=-1
      settings: AttributesFormatString=%<g_funcname>  SourceProductName=Dare Library
  DrMtr_MemoryLengthReqPosi : DareLib/Dare/getAPI_type  g_funcname=Rte_GetVfb_DrMemLengthReqPosi  g_param=""  g_type=uint16  g_size=-1
      settings: AttributesFormatString=%<g_funcname>  SourceProductName=Dare Library
  DrMtr_PowerModeStatus : DareLib/Dare/getAPI_type  g_funcname=Rte_GetVfb_PowerMode  g_param=""  g_type=uint8  g_enum=enIgnSts  g_size=-1
      settings: AttributesFormatString=%<g_funcname>  SourceProductName=Dare Library
  DrMtr_ResBackReqPosi : DareLib/Dare/getAPI_type  g_funcname=Rte_GetVfb_DrResBackReqPosi  g_param=""  g_type=uint16  g_size=-1
      settings: AttributesFormatString=%<g_funcname>  SourceProductName=Dare Library
  DrMtr_ResFrontReqPosi : DareLib/Dare/getAPI_type  g_funcname=Rte_GetVfb_DrResFrontReqPosi  g_param=""  g_type=uint16  g_size=-1
      settings: AttributesFormatString=%<g_funcname>  SourceProductName=Dare Library
  DrMtr_ResHeightReqPosi : DareLib/Dare/getAPI_type  g_funcname=Rte_GetVfb_DrResHeightReqPosi  g_param=""  g_type=uint16  g_size=-1
      settings: AttributesFormatString=%<g_funcname>  SourceProductName=Dare Library
  DrMtr_ResLengthReqPosi : DareLib/Dare/getAPI_type  g_funcname=Rte_GetVfb_DrResLengthReqPosi  g_param=""  g_type=uint16  g_size=-1
      settings: AttributesFormatString=%<g_funcname>  SourceProductName=Dare Library
  DrMtr_ResetBackReqPosi : DareLib/Dare/getAPI_type  g_funcname=Rte_GetVfb_DrBackResetReqPosi  g_param=""  g_type=uint16  g_size=-1
      settings: AttributesFormatString=%<g_funcname>  SourceProductName=Dare Library
  DrMtr_ResetFrontReqPosi : DareLib/Dare/getAPI_type  g_funcname=Rte_GetVfb_DrFrontResetReqPosi  g_param=""  g_type=uint16  g_size=-1
      settings: AttributesFormatString=%<g_funcname>  SourceProductName=Dare Library
  DrMtr_ResetHeightReqPosi : DareLib/Dare/getAPI_type  g_funcname=Rte_GetVfb_DrHeightResetReqPosi  g_param=""  g_type=uint16  g_size=-1
      settings: AttributesFormatString=%<g_funcname>  SourceProductName=Dare Library
  DrMtr_ResetLengthReqPosi : DareLib/Dare/getAPI_type  g_funcname=Rte_GetVfb_DrLengthResetReqPosi  g_param=""  g_type=uint16  g_size=-1
      settings: AttributesFormatString=%<g_funcname>  SourceProductName=Dare Library
  DrMtr_VoltMode : DareLib/Dare/getAPI_type  g_funcname=Rte_GetVfb_VoltMode  g_param=""  g_type=uint8  g_enum=enFinalPowerMode  g_size=-1
      settings: AttributesFormatString=%<g_funcname>  SourceProductName=Dare Library
  DrMtr_VoltSatisfy : DareLib/Dare/getAPI_type  g_funcname=Rte_GetVfb_VoltSatisfy  g_param=""  g_type=uint8  g_size=-1
      settings: AttributesFormatString=%<g_funcname>  SourceProductName=Dare Library
  DrMtr_WelcomeBackReqPosi : DareLib/Dare/getAPI_type  g_funcname=Rte_GetVfb_DrWelBackReqPosi  g_param=""  g_type=uint16  g_size=-1
      settings: AttributesFormatString=%<g_funcname>  SourceProductName=Dare Library
  DrMtr_WelcomeLengthReqPosi : DareLib/Dare/getAPI_type  g_funcname=Rte_GetVfb_DrWelLengthReqPosi  g_param=""  g_type=uint16  g_size=-1
      settings: AttributesFormatString=%<g_funcname>  SourceProductName=Dare Library
  RTE_Signal : Outport
  wires:
  Bus Creator/1 -> RTE_Signal/1  "RTE_Signal"
  DrMtr_ResBackReqPosi/1 -> Bus Creator/15  "DrMtr_ResBackReqPosi"
  DrMtr_ResLengthReqPosi/1 -> Bus Creator/14  "DrMtr_ResLengthReqPosi"
  DrMtr_ResFrontReqPosi/1 -> Bus Creator/16  "DrMtr_ResFrontReqPosi"
  DrMtr_ResHeightReqPosi/1 -> Bus Creator/13  "DrMtr_ResHeightReqPosi"
  DrMtr_ResetHeightReqPosi/1 -> Bus Creator/17  "DrMtr_ResetHeightReqPosi"
  DrMtr_MemoryFrontReqPosi/1 -> Bus Creator/12  "DrMtr_MemoryFrontReqPosi"
  DrMtr_ResetLengthReqPosi/1 -> Bus Creator/18  "DrMtr_ResetLengthReqPosi"
  DrMtr_MemoryBackReqPosi/1 -> Bus Creator/11  "DrMtr_MemoryBackReqPosi"
  DrMtr_ResetBackReqPosi/1 -> Bus Creator/19  "DrMtr_ResetBackReqPosi"
  DrMtr_MemoryLengthReqPosi/1 -> Bus Creator/10  "DrMtr_MemoryLengthReqPosi"
  DrMtr_ResetFrontReqPosi/1 -> Bus Creator/20  "DrMtr_ResetFrontReqPosi"
  DrMtr_MemoryHeightReqPosi/1 -> Bus Creator/9  "DrMtr_MemoryHeightReqPosi"
  DrMtr_WelcomeLengthReqPosi/1 -> Bus Creator/21  "DrMtr_WelcomeLengthReqPosi"
  DrMtr_FrontLearnCmd/1 -> Bus Creator/8  "DrMtr_FrontLearnCmd"
  DrMtr_WelcomeBackReqPosi/1 -> Bus Creator/22  "DrMtr_WelcomeBackReqPosi"
  DrMtr_BackLearnCmd/1 -> Bus Creator/7  "DrMtr_BackLearnCmd"
  DrMtr_DiagnoseLearnIn/1 -> Bus Creator/23  "DrMtr_DiagnoseLearnIn"
  DrMtr_LengthLearnCmd/1 -> Bus Creator/6  "DrMtr_LengthLearnCmd"
  DrMtr_LearnSts/1 -> Bus Creator/24  "DrMtr_LearnSts"
  DrMtr_HeightLearnCmd/1 -> Bus Creator/5  "DrMtr_HeightLearnCmd"
  DrMtr_HeightHallPosi/1 -> Bus Creator/25  "DrMtr_HeightHallPosi"
  DrMtr_FrontSwitchCmd/1 -> Bus Creator/4  "DrMtr_FrontSwitchCmd"
  DrMtr_LengthHallPosi/1 -> Bus Creator/26  "DrMtr_LengthHallPosi"
  DrMtr_BackSwitchCmd/1 -> Bus Creator/3  "DrMtr_BackSwitchCmd"
  DrMtr_BackHallPosi/1 -> Bus Creator/27  "DrMtr_BackHallPosi"
  DrMtr_LengthSwitchCmd/1 -> Bus Creator/2  "DrMtr_LengthSwitchCmd"
  DrMtr_FrontHallPosi/1 -> Bus Creator/28  "DrMtr_FrontHallPosi"
  DrMtr_HeightSwitchCmd/1 -> Bus Creator/1  "DrMtr_HeightSwitchCmd"
  DrMtr_HeightDefaultStopPos/1 -> Bus Creator/29  "DrMtr_HeightDefaultStopPos"
  DrMtr_LengthDefaultStopPos/1 -> Bus Creator/30  "DrMtr_LengthDefaultStopPos"
  DrMtr_BackDefaultStopPos/1 -> Bus Creator/31  "DrMtr_BackDefaultStopPos"
  DrMtr_FrontDefaulStoptPos/1 -> Bus Creator/32  "DrMtr_FrontDefaulStoptPos"
  DrMtr_HeightHallErr/1 -> Bus Creator/33  "DrMtr_HeightHallErr"
  DrMtr_LengthHallErr/1 -> Bus Creator/34  "DrMtr_LengthHallErr"
  DrMtr_BackHallErr/1 -> Bus Creator/35  "DrMtr_BackHallErr"
  DrMtr_FrontHallErr/1 -> Bus Creator/36  "DrMtr_FrontHallErr"
  DrMtr_HeightRelayAdhesionErr/1 -> Bus Creator/37  "DrMtr_HeightRelayAdhesionErr"
  DrMtr_LengthRelayAdhesionErr/1 -> Bus Creator/38  "DrMtr_LengthRelayAdhesionErr"
  DrMtr_BackRelayAdhesionErr/1 -> Bus Creator/39  "DrMtr_BackRelayAdhesionErr"
  DrMtr_FrontRelayAdhesionErr/1 -> Bus Creator/40  "DrMtr_FrontRelayAdhesionErr"
  DrMtr_HeightSwitchAdheErr/1 -> Bus Creator/41  "DrMtr_HeightSwitchAdheErr"
  DrMtr_LengthSwitchAdheErr/1 -> Bus Creator/42  "DrMtr_LengthSwitchAdheErr"
  DrMtr_BackSwitchAdheErr/1 -> Bus Creator/43  "DrMtr_BackSwitchAdheErr"
  DrMtr_FrontSwitchAdheErr/1 -> Bus Creator/44  "DrMtr_FrontSwitchAdheErr"
  DrMtr_HeightStallErr/1 -> Bus Creator/45  "DrMtr_HeightStallErr"
  DrMtr_LengthStallErr/1 -> Bus Creator/46  "DrMtr_LengthStallErr"
  DrMtr_BackStallErr/1 -> Bus Creator/47  "DrMtr_BackStallErr"
  DrMtr_FrontStallErr/1 -> Bus Creator/48  "DrMtr_FrontStallErr"
  DrMtr_AnyoneHallErr/1 -> Bus Creator/49  "DrMtr_AnyoneHallErr"
  DrMtr_AnyoneRelayAdheErr/1 -> Bus Creator/50  "DrMtr_AnyoneRelayAdheErr"
  DrMtr_HeightSoftStopErr/1 -> Bus Creator/51  "DrMtr_HeightSoftStopErr"
  DrMtr_LengthSoftStopErr/1 -> Bus Creator/52  "DrMtr_LengthSoftStopErr"
  DrMtr_BackSoftStopErr/1 -> Bus Creator/53  "DrMtr_BackSoftStopErr"
  DrMtr_FrontSoftStopErr/1 -> Bus Creator/54  "DrMtr_FrontSoftStopErr"
  DrMtr_HeightMotorTimeOutErr/1 -> Bus Creator/55  "DrMtr_HeightMotorTimeOutErr"
  DrMtr_LengthMotorTimeOutErr/1 -> Bus Creator/56  "DrMtr_LengthMotorTimeOutErr"
  DrMtr_BackMotorTimeOutErr/1 -> Bus Creator/57  "DrMtr_BackMotorTimeOutErr"
  DrMtr_FrontMotorTimeOutErr/1 -> Bus Creator/58  "DrMtr_FrontMotorTimeOutErr"
  DrMtr_PowerModeStatus/1 -> Bus Creator/59  "DrMtr_PowerModeStatus"
  DrMtr_VoltMode/1 -> Bus Creator/60  "DrMtr_VoltMode"
  DrMtr_VoltSatisfy/1 -> Bus Creator/61  "DrMtr_VoltSatisfy"
  DrMtr_HeigthMotorMosErr/1 -> Bus Creator/62  "DrMtr_HeigthMotorMosErr"
  DrMtr_LengthMotorMosErr/1 -> Bus Creator/63  "DrMtr_LengthMotorMosErr"
  DrMtr_BackMotorMosErr/1 -> Bus Creator/64  "DrMtr_BackMotorMosErr"
  DrMtr_FrontMotorMosErr/1 -> Bus Creator/65  "DrMtr_FrontMotorMosErr"

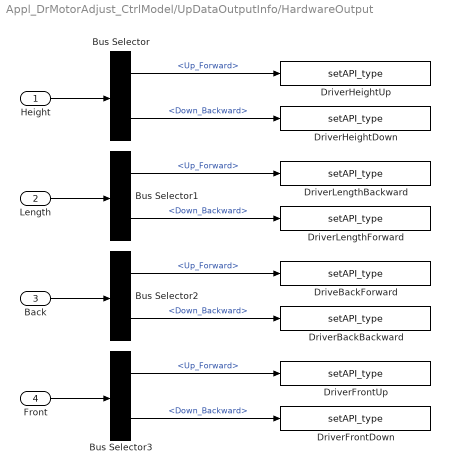
== system Appl_DrMotorAdjust_CtrlModel/UpDataOutputInfo/HardwareOutput ==
  Height : Inport
  Length : Inport  Port=2
  Back : Inport  Port=3
  Front : Inport  Port=4
  Bus Selector{,1..3} (4 alike) : BusSelector  OutputSignals=Up_Forward,Down_Backward
  DriveBackForward : DareLib/Dare/setAPI_type  g_funcname=Ecual_GpioWriteCh  g_param=EN_MCU_PIN6_RELAY_DRV  g_type=uint8  g_size=-1
      settings: AttributesFormatString=%<g_funcname>  SourceProductName=Dare Library
  DriverBackBackward : DareLib/Dare/setAPI_type  g_funcname=Ecual_GpioWriteCh  g_param=EN_MCU_PIN7_RELAY_DRV  g_type=uint8  g_size=-1
      settings: AttributesFormatString=%<g_funcname>  SourceProductName=Dare Library
  DriverFrontDown : DareLib/Dare/setAPI_type  g_funcname=Ecual_GpioWriteCh  g_param=EN_MCU_PIN4_RELAY_DRV  g_type=uint8  g_size=-1
      settings: AttributesFormatString=%<g_funcname>  SourceProductName=Dare Library
  DriverFrontUp : DareLib/Dare/setAPI_type  g_funcname=Ecual_GpioWriteCh  g_param=EN_MCU_PIN9_RELAY_DRV  g_type=uint8  g_size=-1
      settings: AttributesFormatString=%<g_funcname>  SourceProductName=Dare Library
  DriverHeightDown : DareLib/Dare/setAPI_type  g_funcname=Ecual_GpioWriteCh  g_param=EN_MCU_PIN1_RELAY_DRV  g_type=uint8  g_size=-1
      settings: AttributesFormatString=%<g_funcname>  SourceProductName=Dare Library
  DriverHeightUp : DareLib/Dare/setAPI_type  g_funcname=Ecual_GpioWriteCh  g_param=EN_MCU_PIN2_RELAY_DRV  g_type=uint8  g_size=-1
      settings: AttributesFormatString=%<g_funcname>  SourceProductName=Dare Library
  DriverLengthBackward : DareLib/Dare/setAPI_type  g_funcname=Ecual_GpioWriteCh  g_param=EN_MCU_PIN8_RELAY_DRV  g_type=uint8  g_size=-1
      settings: AttributesFormatString=%<g_funcname>  SourceProductName=Dare Library
  DriverLengthForward : DareLib/Dare/setAPI_type  g_funcname=Ecual_GpioWriteCh  g_param=EN_MCU_PIN3_RELAY_DRV  g_type=uint8  g_size=-1
      settings: AttributesFormatString=%<g_funcname>  SourceProductName=Dare Library
  wires:
  Height/1 -> Bus Selector/1
  Bus Selector/1 -> DriverHeightUp/1  "<Up_Forward>"
  Bus Selector/2 -> DriverHeightDown/1  "<Down_Backward>"
  Length/1 -> Bus Selector1/1
  Bus Selector1/1 -> DriverLengthBackward/1  "<Up_Forward>"
  Bus Selector1/2 -> DriverLengthForward/1  "<Down_Backward>"
  Back/1 -> Bus Selector2/1
  Bus Selector2/1 -> DriveBackForward/1  "<Up_Forward>"
  Bus Selector2/2 -> DriverBackBackward/1  "<Down_Backward>"
  Front/1 -> Bus Selector3/1
  Bus Selector3/1 -> DriverFrontUp/1  "<Up_Forward>"
  Bus Selector3/2 -> DriverFrontDown/1  "<Down_Backward>"

== system Appl_DrMotorAdjust_CtrlModel/LogicCtrl/LocalAdjustCtrl/AdjustRequestPriority ==
  MotorReq : Inport
  Bus Selector3 : BusSelector  OutputSignals=HarSwitchCmd.DrMtr_HeightSwitchCmd,HarSwitchCmd.DrMtr_LengthSwitchCmd,HarSwitchCmd.DrMtr_BackSwitchCmd,HarSwitchCmd.DrMtr_FrontSwitchCmd,MemoryReq.DrMtr_MemoryHeightReqPosi,MemoryReq.DrMtr_MemoryLengthReqPosi,MemoryReq.DrMtr_MemoryBackReqPosi,MemoryReq.DrMtr_MemoryFrontReqPosi,ResReq.DrMtr_ResHeightReqPosi,ResReq.DrMtr_ResLengthReqPosi,ResReq.DrMtr_ResBackReqPosi,ResReq.DrMtr_ResFrontReqPosi,WelcomeReq.DrMtr_WelcomeLengthReqPosi,WelcomeReq.DrMtr_WelcomeBackReqPosi,LearnReq.DrMtr_HeightLearnCmd,LearnReq.DrMtr_LengthLearnCmd,LearnReq.DrMtr_BackLearnCmd,LearnReq.DrMtr_FrontLearnCmd,ResetReq.DrMtr_ResetHeightReqPosi,ResetReq.DrMtr_ResetLengthReqPosi,ResetReq.DrMtr_ResetBackReqPosi,ResetReq.DrMtr_ResetFrontReqPosi
  MotorAdjustmentPriorityProcessing1 : Stateflow chart  TreatAsAtomicUnit=on
  setAPI_type : DareLib/Dare/setAPI_type  Commented=on  g_funcname=Srvl_Set_D_SimuIndex_TestValue2  g_param=D_SimuIndex_TestValue2  g_type=uint8  g_size=-1
      settings: AttributesFormatString=%<g_funcname>  SourceProductName=Dare Library
  MotorActType : Outport
  SeatHeightPosiReq : Outport  Port=2
  SeatLengthPosiReq : Outport  Port=3
  SeatBackPosiReq : Outport  Port=4
  SeatFrontPosiReq : Outport  Port=5
  HeightManualAdjSw : Outport  Port=6
  LengthManualAdjSw : Outport  Port=7
  BackManualAdjSw : Outport  Port=8
  FrontManualAdjSw : Outport  Port=9
  wires:
  MotorAdjustmentPriorityProcessing1/1(MotorActionType) -> MotorActType/1
  MotorAdjustmentPriorityProcessing1/2(SeatHeightPosiReq) -> SeatHeightPosiReq/1
  MotorAdjustmentPriorityProcessing1/3(SeatLengthPosiReq) -> SeatLengthPosiReq/1
  MotorAdjustmentPriorityProcessing1/4(SeatBackPosiReq) -> SeatBackPosiReq/1
  MotorAdjustmentPriorityProcessing1/5(SeatFrontPosiReq) -> SeatFrontPosiReq/1
  MotorAdjustmentPriorityProcessing1/6(HeightManualAdjSw) -> HeightManualAdjSw/1
  MotorAdjustmentPriorityProcessing1/7(LengthManualAdjSw) -> LengthManualAdjSw/1
  MotorAdjustmentPriorityProcessing1/8(BackManualAdjSw) -> BackManualAdjSw/1
  MotorAdjustmentPriorityProcessing1/9(FrontManualAdjSw) -> FrontManualAdjSw/1
  MotorAdjustmentPriorityProcessing1/10(TestValue2) -> setAPI_type/1
  MotorReq/1 -> Bus Selector3/1
  Bus Selector3/7 -> MotorAdjustmentPriorityProcessing1/7(DrMtr_MemoryBackReqPosi)  "<DrMtr_MemoryBackReqPosi>"
  Bus Selector3/6 -> MotorAdjustmentPriorityProcessing1/6(DrMtr_MemoryLengthReqPosi)  "<DrMtr_MemoryLengthReqPosi>"
  Bus Selector3/8 -> MotorAdjustmentPriorityProcessing1/8(DrMtr_MemoryFrontReqPosi)  "<DrMtr_MemoryFrontReqPosi>"
  Bus Selector3/5 -> MotorAdjustmentPriorityProcessing1/5(DrMtr_MemoryHeightReqPosi)  "<DrMtr_MemoryHeightReqPosi>"
  Bus Selector3/9 -> MotorAdjustmentPriorityProcessing1/9(DrMtr_ResHeightReqPosi)  "<DrMtr_ResHeightReqPosi>"
  Bus Selector3/4 -> MotorAdjustmentPriorityProcessing1/4(DrMtr_FrontSwitchCmd)  "<DrMtr_FrontSwitchCmd>"
  Bus Selector3/10 -> MotorAdjustmentPriorityProcessing1/10(DrMtr_ResLengthReqPosi)  "<DrMtr_ResLengthReqPosi>"
  Bus Selector3/3 -> MotorAdjustmentPriorityProcessing1/3(DrMtr_BackSwitchCmd)  "<DrMtr_BackSwitchCmd>"
  Bus Selector3/11 -> MotorAdjustmentPriorityProcessing1/11(DrMtr_ResBackReqPosi)  "<DrMtr_ResBackReqPosi>"
  Bus Selector3/2 -> MotorAdjustmentPriorityProcessing1/2(DrMtr_LengthSwitchCmd)  "<DrMtr_LengthSwitchCmd>"
  Bus Selector3/12 -> MotorAdjustmentPriorityProcessing1/12(DrMtr_ResFrontReqPosi)  "<DrMtr_ResFrontReqPosi>"
  Bus Selector3/1 -> MotorAdjustmentPriorityProcessing1/1(DrMtr_HeightSwitchCmd)  "<DrMtr_HeightSwitchCmd>"
  Bus Selector3/13 -> MotorAdjustmentPriorityProcessing1/13(DrMtr_WelcomeLengthReqPosi)  "<DrMtr_WelcomeLengthReqPosi>"
  Bus Selector3/14 -> MotorAdjustmentPriorityProcessing1/14(DrMtr_WelcomeBackReqPosi)  "<DrMtr_WelcomeBackReqPosi>"
  Bus Selector3/15 -> MotorAdjustmentPriorityProcessing1/15(DrMtr_HeightLearnCmd)  "<DrMtr_HeightLearnCmd>"
  Bus Selector3/16 -> MotorAdjustmentPriorityProcessing1/16(DrMtr_LengthLearnCmd)  "<DrMtr_LengthLearnCmd>"
  Bus Selector3/17 -> MotorAdjustmentPriorityProcessing1/17(DrMtr_BackLearnCmd)  "<DrMtr_BackLearnCmd>"
  Bus Selector3/18 -> MotorAdjustmentPriorityProcessing1/18(DrMtr_FrontLearnCmd)  "<DrMtr_FrontLearnCmd>"
  Bus Selector3/19 -> MotorAdjustmentPriorityProcessing1/19(DrMtr_ResetHeightReqPosi)  "<DrMtr_ResetHeightReqPosi>"
  Bus Selector3/20 -> MotorAdjustmentPriorityProcessing1/20(DrMtr_ResetLengthReqPosi)  "<DrMtr_ResetLengthReqPosi>"
  Bus Selector3/21 -> MotorAdjustmentPriorityProcessing1/21(DrMtr_ResetBackReqPosi)  "<DrMtr_ResetBackReqPosi>"
  Bus Selector3/22 -> MotorAdjustmentPriorityProcessing1/22(DrMtr_ResetFrontReqPosi)  "<DrMtr_ResetFrontReqPosi>"

== system Appl_DrMotorAdjust_CtrlModel/LogicCtrl/LocalAdjustCtrl/CrankAndVoltageDeal ==
  CrankAndVoltageDealInput : Inport
  Bus Creator : BusCreator  Inputs=4
  Bus Selector9 : BusSelector  OutputSignals=RteInputBus.Power.DrMtr_PowerModeStatus,RteInputBus.Power.DrMtr_VoltMode,SeatMoveCmd.H_SeatMoveCmd,SeatMoveCmd.L_SeatMoveCmd,SeatMoveCmd.B_SeatMoveCmd,SeatMoveCmd.F_SeatMoveCmd,OTABanFlag,RteInputBus.Power.DrMtr_VoltSatisfy
  CrankUnloading : Stateflow chart  TreatAsAtomicUnit=on
  MotorCmd : Outport
  wires:
  CrankAndVoltageDealInput/1 -> Bus Selector9/1
  Bus Selector9/1 -> CrankUnloading/1(PowerMode)  "<DrMtr_PowerModeStatus>"
  Bus Selector9/2 -> CrankUnloading/2(MtrCtrl_VoltMode)  "<DrMtr_VoltMode>"
  Bus Selector9/3 -> CrankUnloading/3(HeightMotorDirection)  "<H_SeatMoveCmd>"
  Bus Selector9/4 -> CrankUnloading/4(LengthMotorDirection)  "<L_SeatMoveCmd>"
  Bus Selector9/7 -> CrankUnloading/7(DrAdj_OTABanFlag)  "<OTABanFlag>"
  Bus Selector9/8 -> CrankUnloading/8(MtrCtrl_VoltSatisfy)  "<DrMtr_VoltSatisfy>"
  Bus Creator/1 -> MotorCmd/1
  CrankUnloading/1(HeightMotorCmd) -> Bus Creator/1
  CrankUnloading/2(LengthMotorCmd) -> Bus Creator/2
  CrankUnloading/3(BackMotorCmd) -> Bus Creator/3
  CrankUnloading/4(FrontMotorCmd) -> Bus Creator/4
  Bus Selector9/5 -> CrankUnloading/5(BackMotorDirection)  "<B_SeatMoveCmd>"
  Bus Selector9/6 -> CrankUnloading/6(FrontMotorDirection)  "<F_SeatMoveCmd>"
